simulink model "power_elec"  (R2016a)
settings: Solver=ode23tb  StartTime=0.0  StopTime=0.3  MaxStep=1e-5  RelTol=1e-3
libraries: powerlib x12, powerlib_meascontrol x2
settings Model: Creator=Memoir  LastModifiedBy=Memoir
settings DebuggingCC: UnconnectedInputMsg=none  UnconnectedOutputMsg=none  UnconnectedLineMsg=none

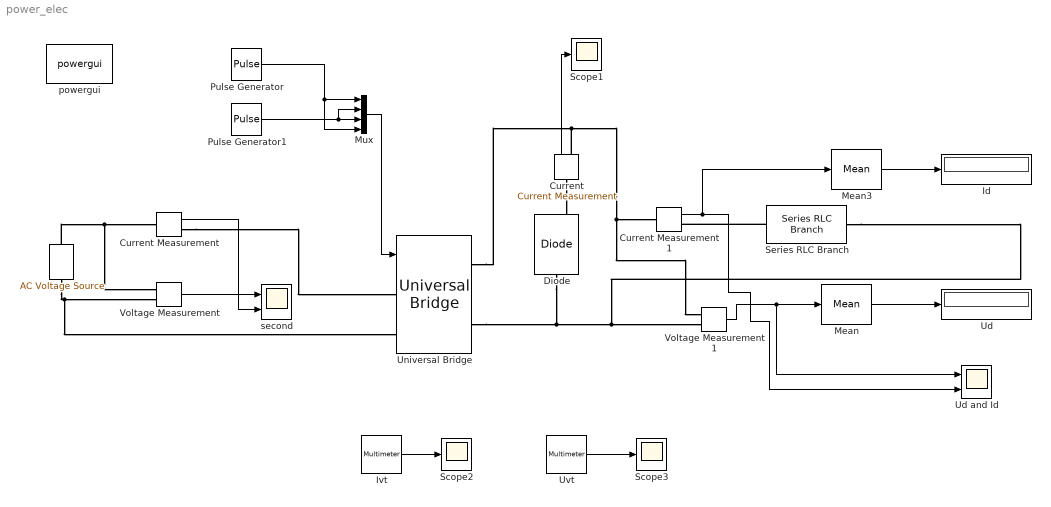
== system power_elec ==
  " " : powerlib/Electrical Sources/AC Voltage Source  Amplitude=220*sqrt(2)  Phase=0  Frequency=50  SampleTime=0  Measurements=None  BusType=swing  Pref=10e3  Qref=0  Qmin=-inf  Qmax=+inf
  Current : powerlib/Measurements/Current Measurement  PhasorSimulation=off  OutputType=Complex  PSBequivalent=0
  Current Measurement : powerlib/Measurements/Current Measurement  PhasorSimulation=off  OutputType=Complex  PSBequivalent=0
  Current Measurement1 : powerlib/Measurements/Current Measurement  PhasorSimulation=off  OutputType=Complex  PSBequivalent=0
  Diode : powerlib/Power Electronics/Diode  Ron=0.001  Lon=0  Vf=0.8  IC=0  UseSnubber=off  Rs=500  Cs=250e-9  Measurements=on
  Id : Display
  Ivt : powerlib/Measurements/Multimeter  PhasorSimulation=off  OutputType=Complex  sel=7  L=10  Gain=1  yselected={'Isw1: Universal Bridge'};  PSBOutputType=1  PSBequivalent=0  AxesSetting=[0,0.1,-100,100]  Display=0  SavedBlockNames=-11
  Mean : powerlib_meascontrol/Measurements/Mean  Freq=50  Vinit=0  Ts=0
  Mean3 : powerlib_meascontrol/Measurements/Mean  Freq=50  Vinit=0  Ts=0
  Mux : Mux
  Pulse Generator : DiscretePulseGenerator  PulseType=Time based  Period=0.02  PulseWidth=10  PhaseDelay=30*0.02/360
  Pulse Generator1 : DiscretePulseGenerator  PulseType=Time based  Period=0.02  PulseWidth=10  PhaseDelay=0.02*30/360+0.01
  Scope1 : Scope
  Scope2 : Scope
  Scope3 : Scope
  Series RLC Branch : powerlib/Elements/Series RLC Branch  LConnTagsString=__new0  RConnTagsString=__new0  BranchType=RL  Resistance=10  Inductance=0.3  SetiL0=off  InitialCurrent=0  Capacitance=1e-6  Setx0=off  InitialVoltage=0  Measurements=None
  Ud : Display
  Ud and Id : Scope  NumInputPorts=2
  Universal Bridge : powerlib/Power Electronics/Universal Bridge  Arms=2  SnubberResistance=1e6  SnubberCapacitance=inf  Device=Thyristors  Ron=1e-3  Lon=0  ForwardVoltages="[  0  0  ]"  ForwardVoltage=0  GTOparameters=[ 10e-6 , 20e-6 ]  IGBTparameters=[ 1e-6 , 2e-6 ]  Measurements=All voltages and currents  Measurements_2=None  converterType=Rectifier
  Uvt : powerlib/Measurements/Multimeter  PhasorSimulation=off  OutputType=Complex  sel=1  L=10  Gain=1  yselected={'Usw1: Universal Bridge'};  PSBOutputType=1  PSBequivalent=0  AxesSetting=[0,0.1,-100,100]  Display=0  SavedBlockNames=-11
  Voltage Measurement : powerlib/Measurements/Voltage Measurement  PhasorSimulation=off  OutputType=Complex  PSBequivalent=0
  Voltage Measurement1 : powerlib/Measurements/Voltage Measurement  PhasorSimulation=off  OutputType=Complex  PSBequivalent=0
  powergui : powerlib/powergui  Priority=1  SimulationMode=Continuous  SolverType=Tustin/Backward Euler (TBE)  SampleTime=50e-6  frequency=60  SPID=on  DisableSnubberDevices=off  DisableRonSwitches=off  DisableVfSwitches=off  SwTol=0  DisplayEquations=off  Interpol=off  ExternalGateDelay=off  methode=off  Ts=10  FunctionMessages=off  echomessages=off  HookPort=off  EnableUseOfTLC=off  x0status=blocks  frequencyindice=50  Pbase=100e6  ErrMax=1e-4  Iterations=50  UnitsV=kV  UnitsW=MW  buscounter=0  RestoreLinks=warning  ResistiveCurrentMeasurement=off  Frange=[0:2:500]  Ylog=off  Xlog=on  ShowGrid=off  save=off  variable=ZData  structure=0  ZoomFFT=off  StartTime=0.0  cycles=1  DisplayStyle=1  fundamental=60  FreqAxis=off  MaxFrequency=1000  frequencyindicesteady=1  RmsSteady=1  display=off
  second : Scope  NumInputPorts=2
  wires:
  Mean/1 -> Ud/1
  Voltage Measurement1/1 -> Ud and Id/1, Mean/1
  Pulse Generator/1 -> Mux/4, Mux/1
  Pulse Generator1/1 -> Mux/2, Mux/3
  Mux/1 -> Universal Bridge/1
  Voltage Measurement/1 -> second/1
  Current Measurement/1 -> second/2
  Uvt/1 -> Scope3/1
  Current/1 -> Scope1/1
  Mean3/1 -> Id/1
  Current Measurement1/1 -> Mean3/1, Ud and Id/2
  Ivt/1 -> Scope2/1
  connections:
  Universal Bridge/RConn2 -- Diode/LConn1 -- Series RLC Branch/RConn1 -- Voltage Measurement1/LConn2
  Series RLC Branch/LConn1 -- Current Measurement1/RConn1
  Universal Bridge/RConn1 -- Current/RConn1 -- Voltage Measurement1/LConn1 -- Current Measurement1/LConn1
  " "/RConn1 -- Voltage Measurement/LConn1 -- Current Measurement/LConn1
  " "/LConn1 -- Universal Bridge/LConn2 -- Voltage Measurement/LConn2
  Current Measurement/RConn1 -- Universal Bridge/LConn1
  Current/LConn1 -- Diode/RConn1
